simulink model "Lorenz_Simulink"  (R2021a)
settings: Solver=VariableStepAuto  StartTime=0.0  StopTime=10.0  RelTol=1e-3
settings Model: Creator=Marcial  LastModifiedBy=Marcial

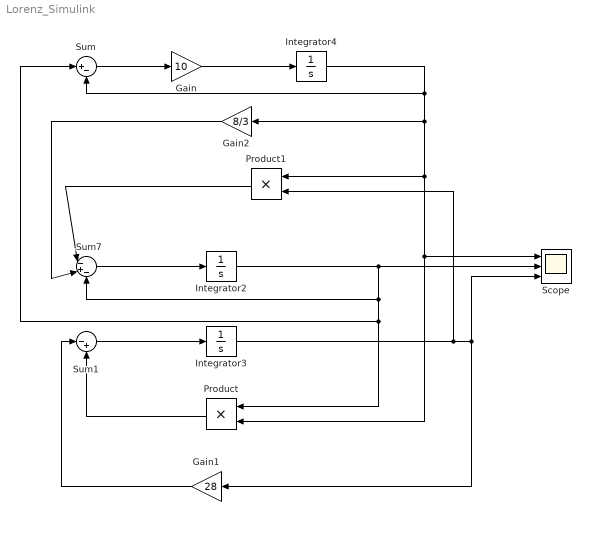
== system Lorenz_Simulink ==
  Gain : Gain  Gain=10
  Gain1 : Gain  Gain=28
  Gain2 : Gain  Gain=8/3
  Integrator2 : Integrator  InitialCondition=-8
  Integrator3 : Integrator  InitialCondition=24
  Integrator4 : Integrator  InitialCondition=-8
  Product : Product
  Product1 : Product
  Scope : Scope  NumInputPorts=3
  Sum : Sum  Inputs=|+-
  Sum1 : Sum  Inputs=|-+
  Sum7 : Sum  Inputs=|-+-
  wires:
  Sum1/1 -> Integrator3/1
  Product/1 -> Sum1/2
  Gain1/1 -> Sum1/1
  Integrator3/1 -> Product1/2, Scope/3, Gain1/1
  Integrator2/1 -> Sum7/3, Sum/1, Product/1, Scope/2
  Sum7/1 -> Integrator2/1
  Gain/1 -> Integrator4/1
  Gain2/1 -> Sum7/2
  Product1/1 -> Sum7/1
  Sum/1 -> Gain/1
  Integrator4/1 -> Scope/1, Product/2, Product1/1, Gain2/1, Sum/2
